simulink model "AGTF30PwrSys"  (R2021b)
settings: Solver=FixedStepDiscrete  StartTime=0.0  StopTime=MWS.In.tend  RelTol=1e-3
values from neighbouring files (symbols this model uses):
  MWS = setup_initialize(MWS,startPt,SSsolverSP)    [Setup_Simulation.m]    (also in run_AGTF30e_script.m = Setup_Simulation(inputMethod,MWS.In,filename,Mdl,SSsolverSP,)
settings Model: Creator=jlkratz  LastModifiedBy=jlkratz
settings SolverCC: ZeroCrossControl=DisableAll  AlgebraicLoopSolver=TrustRegion
settings DataIOCC: SaveOutput=off  SaveTime=off
settings DebuggingCC: SFMachineParentedDataDiag=warning
settings GRTTargetCC: CombineOutputUpdateFcns=off  MatFileLogging=off

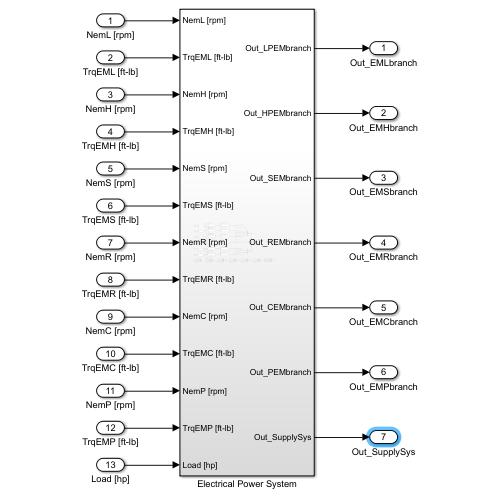
[thumbnail: Simulink's stored preview of the top-level diagram]
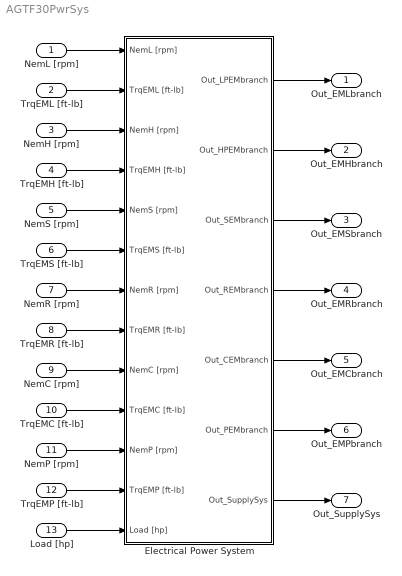
== system AGTF30PwrSys ==
  NemL [rpm] : Inport
  TrqEML [ft-lb] : Inport  Port=2
  NemH [rpm] : Inport  Port=3
  TrqEMH [ft-lb] : Inport  Port=4
  NemS [rpm] : Inport  Port=5
  TrqEMS [ft-lb] : Inport  Port=6
  NemR [rpm] : Inport  Port=7
  TrqEMR [ft-lb] : Inport  Port=8
  NemC [rpm] : Inport  Port=9
  TrqEMC [ft-lb] : Inport  Port=10
  NemP [rpm] : Inport  Port=11
  TrqEMP [ft-lb] : Inport  Port=12
  Load [hp] : Inport  Port=13
  Electrical Power System : Subsystem
  Out_EMLbranch : Outport
  Out_EMHbranch : Outport  Port=2
  Out_EMSbranch : Outport  Port=3
  Out_EMRbranch : Outport  Port=4
  Out_EMCbranch : Outport  Port=5
  Out_EMPbranch : Outport  Port=6
  Out_SupplySys : Outport  Port=7
  wires:
  NemL [rpm]/1 -> Electrical Power System/1(NemL [rpm])
  TrqEML [ft-lb]/1 -> Electrical Power System/2(TrqEML [ft-lb])
  NemH [rpm]/1 -> Electrical Power System/3(NemH [rpm])
  TrqEMH [ft-lb]/1 -> Electrical Power System/4(TrqEMH [ft-lb])
  Electrical Power System/1(Out_LPEMbranch) -> Out_EMLbranch/1
  Electrical Power System/2(Out_HPEMbranch) -> Out_EMHbranch/1
  Electrical Power System/7(Out_SupplySys) -> Out_SupplySys/1
  NemS [rpm]/1 -> Electrical Power System/5(NemS [rpm])
  TrqEMS [ft-lb]/1 -> Electrical Power System/6(TrqEMS [ft-lb])
  NemR [rpm]/1 -> Electrical Power System/7(NemR [rpm])
  TrqEMR [ft-lb]/1 -> Electrical Power System/8(TrqEMR [ft-lb])
  NemC [rpm]/1 -> Electrical Power System/9(NemC [rpm])
  TrqEMC [ft-lb]/1 -> Electrical Power System/10(TrqEMC [ft-lb])
  NemP [rpm]/1 -> Electrical Power System/11(NemP [rpm])
  TrqEMP [ft-lb]/1 -> Electrical Power System/12(TrqEMP [ft-lb])
  Load [hp]/1 -> Electrical Power System/13(Load [hp])
  Electrical Power System/3(Out_SEMbranch) -> Out_EMSbranch/1
  Electrical Power System/4(Out_REMbranch) -> Out_EMRbranch/1
  Electrical Power System/5(Out_CEMbranch) -> Out_EMCbranch/1
  Electrical Power System/6(Out_PEMbranch) -> Out_EMPbranch/1

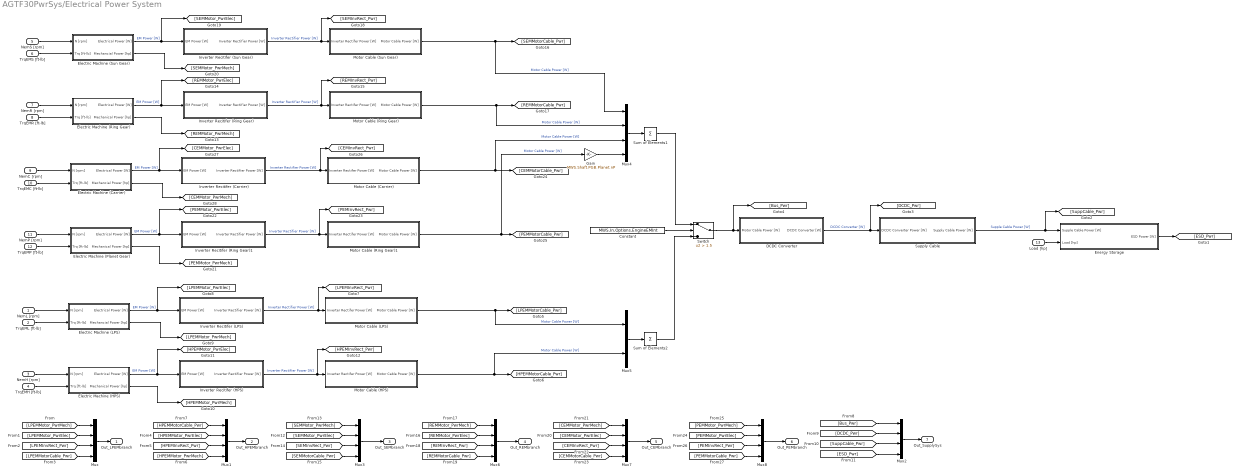
== system AGTF30PwrSys/Electrical Power System ==
  NemL [rpm] : Inport
  TrqEML [ft-lb] : Inport  Port=2
  NemH [rpm] : Inport  Port=3
  TrqEMH [ft-lb] : Inport  Port=4
  NemS [rpm] : Inport  Port=5
  TrqEMS [ft-lb] : Inport  Port=6
  NemR [rpm] : Inport  Port=7
  TrqEMR [ft-lb] : Inport  Port=8
  NemC [rpm] : Inport  Port=9
  TrqEMC [ft-lb] : Inport  Port=10
  NemP [rpm] : Inport  Port=11
  TrqEMP [ft-lb] : Inport  Port=12
  Load [hp] : Inport  Port=13
  Constant : Constant  Value=MWS.In.Options.EngineEMInt
  DCDC Converter : Subsystem
  Electric Machine (Carrier) : Subsystem
  Electric Machine (HPS) : Subsystem
  Electric Machine (LPS) : Subsystem
  Electric Machine (Planet Gear) : Subsystem
  Electric Machine (Ring Gear) : Subsystem
  Electric Machine (Sun Gear) : Subsystem
  Energy Storage : Subsystem
  Gain : Gain  Gain=MWS.Shaft.PGB.Planet.nP
  Inverter Recitifer (Carrier) : Subsystem
  Inverter Recitifer (HPS) : Subsystem
  Inverter Recitifer (LPS) : Subsystem
  Inverter Recitifer (Ring Gear) : Subsystem
  Inverter Recitifer (Ring Gear)1 : Subsystem
  Inverter Recitifer (Sun Gear) : Subsystem
  Motor Cable (Carrier) : Subsystem
  Motor Cable (HPS) : Subsystem
  Motor Cable (LPS) : Subsystem
  Motor Cable (Ring Gear) : Subsystem
  Motor Cable (Ring Gear)1 : Subsystem
  Motor Cable (Sun Gear) : Subsystem
  Mux{,1..4,6..8} (8 alike) : Mux
  Mux5 : Mux  Inputs=2
  Sum of Elements1 : Sum  Inputs=+
  Sum of Elements2 : Sum  Inputs=+
  "Supply Cable " : Subsystem
  Switch : Switch  Criteria=u2 > Threshold  Threshold=1.5
  Out_LPEMbranch : Outport
  Out_HPEMbranch : Outport  Port=2
  Out_SEMbranch : Outport  Port=3
  Out_REMbranch : Outport  Port=4
  Out_CEMbranch : Outport  Port=5
  Out_PEMbranch : Outport  Port=6
  Out_SupplySys : Outport  Port=7
  wires:
  Motor Cable (LPS)/1(Motor Cable Power [W]) -> Mux5/1, [LPEMMotorCable_Pwr]  "Motor Cable Power [W]"
  Motor Cable (HPS)/1(Motor Cable Power [W]) -> Mux5/2, [HPEMMotorCable_Pwr]  "Motor Cable Power [W]"
  Inverter Recitifer (HPS)/1(Inverter Rectifier Power [W]) -> [HPEMInvRect_Pwr], Motor Cable (HPS)/1(Inverter Rectifer Power [W])  "Inverter Rectifier Power [W]"
  [ESD_Pwr] -> Mux2/4
  "Supply Cable "/1(Supply Cable Power [W]) -> [SuppCable_Pwr], Energy Storage/1(Supple Cable Power [W])  "Supple Cable Power [W]"
  [SuppCable_Pwr] -> Mux2/3
  Electric Machine (HPS)/1(Electrical Power [W]) -> Inverter Recitifer (HPS)/1(EM Power [W]), [HPEMMotor_PwrElec]  "EM Power [W]"
  Mux2/1 -> Out_SupplySys/1
  TrqEML [ft-lb]/1 -> Electric Machine (LPS)/2(Trq [ft-lb])
  NemL [rpm]/1 -> Electric Machine (LPS)/1(N [rpm])
  Mux/1 -> Out_LPEMbranch/1
  Electric Machine (HPS)/2(Mechanical Power [hp]) -> [HPEMMotor_PwrMech]
  DCDC Converter/1(DCDC Converter [W]) -> [DCDC_Pwr], "Supply Cable "/1(DCDC Converter Power [W])  "DCDC Converter [W]"
  Inverter Recitifer (LPS)/1(Inverter Rectifier Power [W]) -> [LPEMInvRect_Pwr], Motor Cable (LPS)/1(Inverter Rectifer Power [W])  "Inverter Rectifier Power [W]"
  Switch/1 -> [Bus_Pwr], DCDC Converter/1(Motor Cable Power [W])
  NemH [rpm]/1 -> Electric Machine (HPS)/1(N [rpm])
  Electric Machine (LPS)/1(Electrical Power [W]) -> Inverter Recitifer (LPS)/1(EM Power [W]), [LPEMMotor_PwrElec]  "EM Power [W]"
  Electric Machine (LPS)/2(Mechancial Power [hp]) -> [LPEMMotor_PwrMech]
  Mux1/1 -> Out_HPEMbranch/1
  [Bus_Pwr] -> Mux2/1
  Energy Storage/1(ESD Power [W]) -> [ESD_Pwr]
  TrqEMH [ft-lb]/1 -> Electric Machine (HPS)/2(Trq [ft-lb])
  [DCDC_Pwr] -> Mux2/2
  Load [hp]/1 -> Energy Storage/2(Load [hp])
  TrqEMR [ft-lb]/1 -> Electric Machine (Ring Gear)/2(Trq [ft-lb])
  Electric Machine (Sun Gear)/2(Mechancial Power [hp]) -> [SEMMotor_PwrMech]
  Electric Machine (Sun Gear)/1(Electrical Power [W]) -> [SEMMotor_PwrElec], Inverter Recitifer (Sun Gear)/1(EM Power [W])  "EM Power [W]"
  NemR [rpm]/1 -> Electric Machine (Ring Gear)/1(N [rpm])
  Inverter Recitifer (Sun Gear)/1(Inverter Rectifier Power [W]) -> Motor Cable (Sun Gear)/1(Inverter Rectifer Power [W]), [SEMInvRect_Pwr]  "Inverter Rectifier Power [W]"
  Electric Machine (Ring Gear)/2(Mechanical Power [hp]) -> [REMMotor_PwrMech]
  NemS [rpm]/1 -> Electric Machine (Sun Gear)/1(N [rpm])
  TrqEMS [ft-lb]/1 -> Electric Machine (Sun Gear)/2(Trq [ft-lb])
  Electric Machine (Ring Gear)/1(Electrical Power [W]) -> [REMMotor_PwrElec], Inverter Recitifer (Ring Gear)/1(EM Power [W])  "EM Power [W]"
  Inverter Recitifer (Ring Gear)/1(Inverter Rectifier Power [W]) -> Motor Cable (Ring Gear)/1(Inverter Rectifer Power [W]), [REMInvRect_Pwr]  "Inverter Rectifier Power [W]"
  Motor Cable (Ring Gear)/1(Motor Cable Power [W]) -> Mux4/2, [REMMotorCable_Pwr]  "Motor Cable Power [W]"
  Motor Cable (Sun Gear)/1(Motor Cable Power [W]) -> [SEMMotorCable_Pwr], Mux4/1  "Motor Cable Power [W]"
  Motor Cable (Carrier)/1(Motor Cable Power [W]) -> Mux4/3, [CEMMotorCable_Pwr]  "Motor Cable Power [W]"
  Motor Cable (Ring Gear)1/1(Motor Cable Power [W]) -> [PEMMotorCable_Pwr], Gain/1  "Motor Cable Power [W]"
  Inverter Recitifer (Ring Gear)1/1(Inverter Rectifier Power [W]) -> [PEMInvRect_Pwr], Motor Cable (Ring Gear)1/1(Inverter Rectifer Power [W])  "Inverter Rectifier Power [W]"
  Electric Machine (Planet Gear)/1(Electrical Power [W]) -> Inverter Recitifer (Ring Gear)1/1(EM Power [W]), [PEMMotor_PwrElec]  "EM Power [W]"
  TrqEMC [ft-lb]/1 -> Electric Machine (Carrier)/2(Trq [ft-lb])
  NemC [rpm]/1 -> Electric Machine (Carrier)/1(N [rpm])
  Electric Machine (Planet Gear)/2(Mechanical Power [hp]) -> [PEMMotor_PwrMech]
  Inverter Recitifer (Carrier)/1(Inverter Rectifier Power [W]) -> [CEMInvRect_Pwr], Motor Cable (Carrier)/1(Inverter Rectifer Power [W])  "Inverter Rectifier Power [W]"
  NemP [rpm]/1 -> Electric Machine (Planet Gear)/1(N [rpm])
  Electric Machine (Carrier)/1(Electrical Power [W]) -> Inverter Recitifer (Carrier)/1(EM Power [W]), [CEMMotor_PwrElec]  "EM Power [W]"
  Electric Machine (Carrier)/2(Mechancial Power [hp]) -> [CEMMotor_PwrMech]
  TrqEMP [ft-lb]/1 -> Electric Machine (Planet Gear)/2(Trq [ft-lb])
  Mux4/1 -> Sum of Elements1/1
  Mux5/1 -> Sum of Elements2/1
  Sum of Elements1/1 -> Switch/1
  Sum of Elements2/1 -> Switch/3
  Constant/1 -> Switch/2
  [SEMMotor_PwrMech] -> Mux3/1
  [SEMMotor_PwrElec] -> Mux3/2
  [SEMInvRect_Pwr] -> Mux3/3
  [SEMMotorCable_Pwr] -> Mux3/4
  [LPEMMotor_PwrMech] -> Mux/1
  [LPEMMotor_PwrElec] -> Mux/2
  [LPEMInvRect_Pwr] -> Mux/3
  [LPEMMotorCable_Pwr] -> Mux/4
  [HPEMMotor_PwrElec] -> Mux1/2
  [HPEMInvRect_Pwr] -> Mux1/3
  [HPEMMotor_PwrMech] -> Mux1/4
  [HPEMMotorCable_Pwr] -> Mux1/1
  Mux3/1 -> Out_SEMbranch/1
  Mux6/1 -> Out_REMbranch/1
  [REMMotorCable_Pwr] -> Mux6/4
  [REMInvRect_Pwr] -> Mux6/3
  [REMMotor_PwrElec] -> Mux6/2
  [REMMotor_PwrMech] -> Mux6/1
  [PEMMotor_PwrMech] -> Mux8/1
  [PEMMotor_PwrElec] -> Mux8/2
  [PEMInvRect_Pwr] -> Mux8/3
  [PEMMotorCable_Pwr] -> Mux8/4
  Mux8/1 -> Out_PEMbranch/1
  Mux7/1 -> Out_CEMbranch/1
  [CEMMotorCable_Pwr] -> Mux7/4
  [CEMInvRect_Pwr] -> Mux7/3
  [CEMMotor_PwrElec] -> Mux7/2
  [CEMMotor_PwrMech] -> Mux7/1
  Gain/1 -> Mux4/4

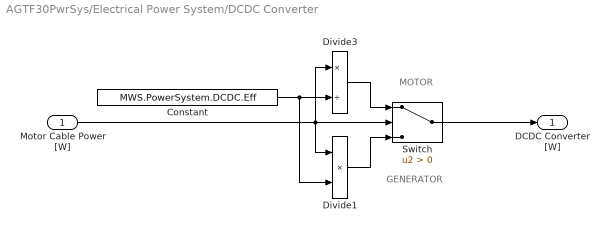
== system AGTF30PwrSys/Electrical Power System/DCDC Converter ==
  note: GENERATOR
  note: MOTOR
  Motor Cable Power [W] : Inport
  Constant : Constant  Value=MWS.PowerSystem.DCDC.Eff
  Divide1 : Product  Inputs=**
  Divide3 : Product  Inputs=*/
  Switch : Switch  Criteria=u2 > Threshold
  DCDC Converter [W] : Outport
  wires:
  Constant/1 -> Divide1/2, Divide3/2
  Switch/1 -> DCDC Converter [W]/1
  Divide3/1 -> Switch/1
  Divide1/1 -> Switch/3
  Motor Cable Power [W]/1 -> Divide3/1, Divide1/1, Switch/2

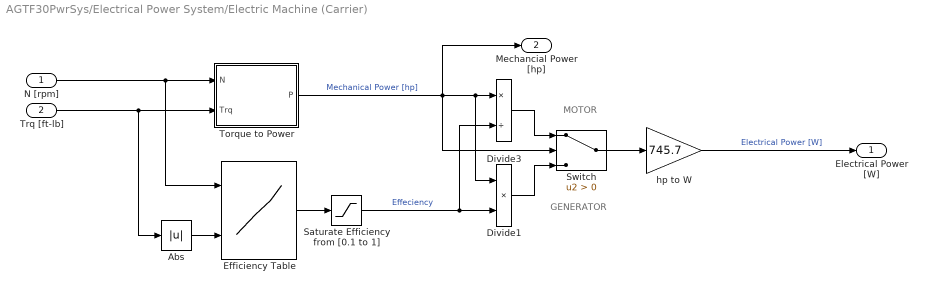
== system AGTF30PwrSys/Electrical Power System/Electric Machine (Carrier) ==
  note: MOTOR
  note: GENERATOR
  N [rpm] : Inport
  Trq [ft-lb] : Inport  Port=2
  Abs : Abs
  Divide1 : Product  Inputs=**
  Divide3 : Product  Inputs=*/
  Efficiency Table : Lookup_n-D  BreakpointsForDimension1=MWS.PowerSystem.EMS.Speed  BreakpointsForDimension2=MWS.PowerSystem.EMS.Torque  Table=MWS.PowerSystem.EMS.Eff  ExtrapMethod=Clip  InternalRulePriority=Speed  RndMeth=Simplest  InputSameDT=on
      settings: InputPortMap=u0,u1
  Saturate Efficiency from [0.1 to 1] : Saturate  UpperLimit=1  LowerLimit=0.1
  Switch : Switch  Criteria=u2 > Threshold
  Torque to Power : Subsystem
  hp to W : Gain  Gain=745.7
  Electrical Power [W] : Outport
  Mechancial Power [hp] : Outport  Port=2
  wires:
  Switch/1 -> hp to W/1
  Saturate Efficiency from [0.1 to 1]/1 -> Divide3/2, Divide1/2  "Effeciency"
  Torque to Power/1(P) -> Mechancial Power [hp]/1, Switch/2, Divide1/1, Divide3/1  "Mechanical Power [hp]"
  Divide1/1 -> Switch/3
  N [rpm]/1 -> Efficiency Table/1, Torque to Power/1(N)
  Efficiency Table/1 -> Saturate Efficiency from [0.1 to 1]/1
  Trq [ft-lb]/1 -> Abs/1, Torque to Power/2(Trq)
  Abs/1 -> Efficiency Table/2
  Divide3/1 -> Switch/1
  hp to W/1 -> Electrical Power [W]/1  "Electrical Power [W]"

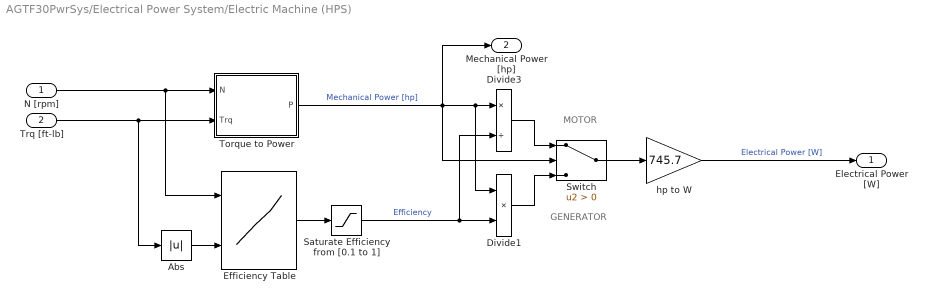
== system AGTF30PwrSys/Electrical Power System/Electric Machine (HPS) ==
  note: GENERATOR
  note: MOTOR
  N [rpm] : Inport
  Trq [ft-lb] : Inport  Port=2
  Abs : Abs
  Divide1 : Product  Inputs=**
  Divide3 : Product  Inputs=*/
  Efficiency Table : Lookup_n-D  BreakpointsForDimension1=MWS.PowerSystem.EMH.Speed  BreakpointsForDimension2=MWS.PowerSystem.EMH.Torque  Table=MWS.PowerSystem.EMH.Eff  ExtrapMethod=Clip  InternalRulePriority=Speed  RndMeth=Simplest  InputSameDT=on
      settings: InputPortMap=u0,u1
  Saturate Efficiency from [0.1 to 1] : Saturate  UpperLimit=1  LowerLimit=0.1
  Switch : Switch  Criteria=u2 > Threshold
  Torque to Power : Subsystem
  hp to W : Gain  Gain=745.7
  Electrical Power [W] : Outport
  Mechanical Power [hp] : Outport  Port=2
  wires:
  hp to W/1 -> Electrical Power [W]/1  "Electrical Power [W]"
  Divide3/1 -> Switch/1
  Abs/1 -> Efficiency Table/2
  Trq [ft-lb]/1 -> Torque to Power/2(Trq), Abs/1
  Efficiency Table/1 -> Saturate Efficiency from [0.1 to 1]/1
  N [rpm]/1 -> Torque to Power/1(N), Efficiency Table/1
  Divide1/1 -> Switch/3
  Torque to Power/1(P) -> Mechanical Power [hp]/1, Divide3/1, Divide1/1, Switch/2  "Mechanical Power [hp]"
  Saturate Efficiency from [0.1 to 1]/1 -> Divide1/2, Divide3/2  "Efficiency"
  Switch/1 -> hp to W/1

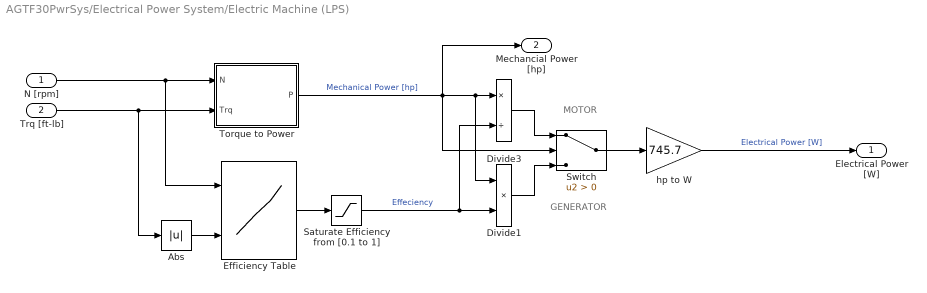
== system AGTF30PwrSys/Electrical Power System/Electric Machine (LPS) ==
  note: MOTOR
  note: GENERATOR
  N [rpm] : Inport
  Trq [ft-lb] : Inport  Port=2
  Abs : Abs
  Divide1 : Product  Inputs=**
  Divide3 : Product  Inputs=*/
  Efficiency Table : Lookup_n-D  BreakpointsForDimension1=MWS.PowerSystem.EML.Speed  BreakpointsForDimension2=MWS.PowerSystem.EML.Torque  Table=MWS.PowerSystem.EML.Eff  ExtrapMethod=Clip  InternalRulePriority=Speed  RndMeth=Simplest  InputSameDT=on
      settings: InputPortMap=u0,u1
  Saturate Efficiency from [0.1 to 1] : Saturate  UpperLimit=1  LowerLimit=0.1
  Switch : Switch  Criteria=u2 > Threshold
  Torque to Power : Subsystem
  hp to W : Gain  Gain=745.7
  Electrical Power [W] : Outport
  Mechancial Power [hp] : Outport  Port=2
  wires:
  Switch/1 -> hp to W/1
  Saturate Efficiency from [0.1 to 1]/1 -> Divide3/2, Divide1/2  "Effeciency"
  Torque to Power/1(P) -> Mechancial Power [hp]/1, Switch/2, Divide1/1, Divide3/1  "Mechanical Power [hp]"
  Divide1/1 -> Switch/3
  N [rpm]/1 -> Efficiency Table/1, Torque to Power/1(N)
  Efficiency Table/1 -> Saturate Efficiency from [0.1 to 1]/1
  Trq [ft-lb]/1 -> Abs/1, Torque to Power/2(Trq)
  Abs/1 -> Efficiency Table/2
  Divide3/1 -> Switch/1
  hp to W/1 -> Electrical Power [W]/1  "Electrical Power [W]"

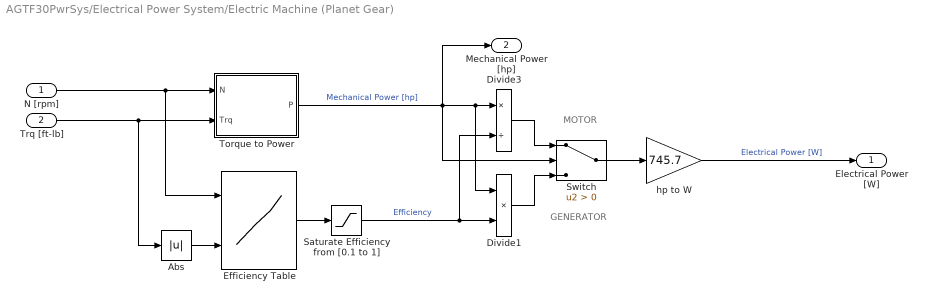
== system AGTF30PwrSys/Electrical Power System/Electric Machine (Planet Gear) ==
  note: GENERATOR
  note: MOTOR
  N [rpm] : Inport
  Trq [ft-lb] : Inport  Port=2
  Abs : Abs
  Divide1 : Product  Inputs=**
  Divide3 : Product  Inputs=*/
  Efficiency Table : Lookup_n-D  BreakpointsForDimension1=MWS.PowerSystem.EMR.Speed  BreakpointsForDimension2=MWS.PowerSystem.EMR.Torque  Table=MWS.PowerSystem.EMR.Eff  ExtrapMethod=Clip  InternalRulePriority=Speed  RndMeth=Simplest  InputSameDT=on
      settings: InputPortMap=u0,u1
  Saturate Efficiency from [0.1 to 1] : Saturate  UpperLimit=1  LowerLimit=0.1
  Switch : Switch  Criteria=u2 > Threshold
  Torque to Power : Subsystem
  hp to W : Gain  Gain=745.7
  Electrical Power [W] : Outport
  Mechanical Power [hp] : Outport  Port=2
  wires:
  hp to W/1 -> Electrical Power [W]/1  "Electrical Power [W]"
  Divide3/1 -> Switch/1
  Abs/1 -> Efficiency Table/2
  Trq [ft-lb]/1 -> Torque to Power/2(Trq), Abs/1
  Efficiency Table/1 -> Saturate Efficiency from [0.1 to 1]/1
  N [rpm]/1 -> Torque to Power/1(N), Efficiency Table/1
  Divide1/1 -> Switch/3
  Torque to Power/1(P) -> Mechanical Power [hp]/1, Divide3/1, Divide1/1, Switch/2  "Mechanical Power [hp]"
  Saturate Efficiency from [0.1 to 1]/1 -> Divide1/2, Divide3/2  "Efficiency"
  Switch/1 -> hp to W/1

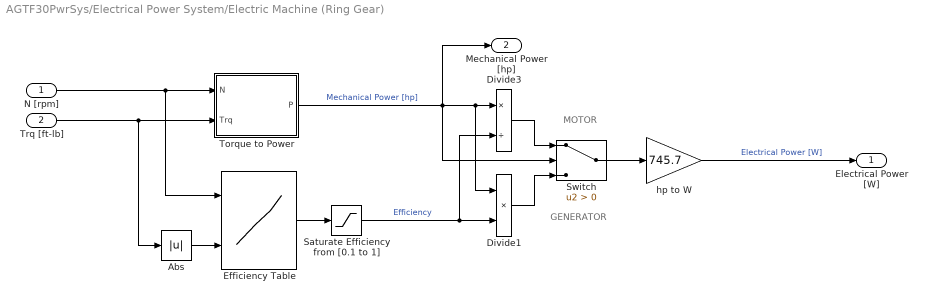
== system AGTF30PwrSys/Electrical Power System/Electric Machine (Ring Gear) ==
  note: MOTOR
  note: GENERATOR
  N [rpm] : Inport
  Trq [ft-lb] : Inport  Port=2
  Abs : Abs
  Divide1 : Product  Inputs=**
  Divide3 : Product  Inputs=*/
  Efficiency Table : Lookup_n-D  BreakpointsForDimension1=MWS.PowerSystem.EMR.Speed  BreakpointsForDimension2=MWS.PowerSystem.EMR.Torque  Table=MWS.PowerSystem.EMR.Eff  ExtrapMethod=Clip  InternalRulePriority=Speed  RndMeth=Simplest  InputSameDT=on
      settings: InputPortMap=u0,u1
  Saturate Efficiency from [0.1 to 1] : Saturate  UpperLimit=1  LowerLimit=0.1
  Switch : Switch  Criteria=u2 > Threshold
  Torque to Power : Subsystem
  hp to W : Gain  Gain=745.7
  Electrical Power [W] : Outport
  Mechanical Power [hp] : Outport  Port=2
  wires:
  Switch/1 -> hp to W/1
  Saturate Efficiency from [0.1 to 1]/1 -> Divide3/2, Divide1/2  "Efficiency"
  Torque to Power/1(P) -> Switch/2, Divide1/1, Divide3/1, Mechanical Power [hp]/1  "Mechanical Power [hp]"
  Divide1/1 -> Switch/3
  N [rpm]/1 -> Efficiency Table/1, Torque to Power/1(N)
  Efficiency Table/1 -> Saturate Efficiency from [0.1 to 1]/1
  Trq [ft-lb]/1 -> Abs/1, Torque to Power/2(Trq)
  Abs/1 -> Efficiency Table/2
  Divide3/1 -> Switch/1
  hp to W/1 -> Electrical Power [W]/1  "Electrical Power [W]"

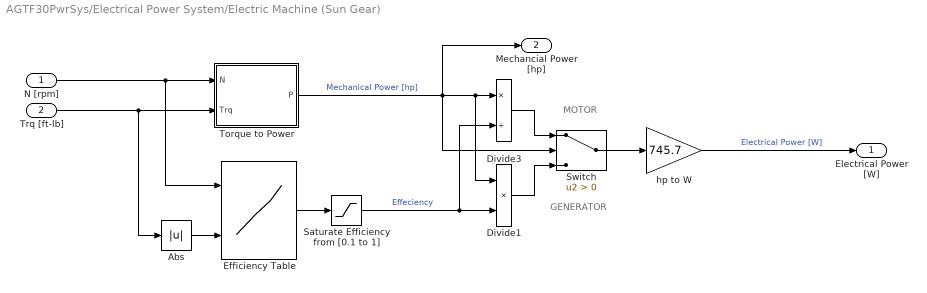
== system AGTF30PwrSys/Electrical Power System/Electric Machine (Sun Gear) ==
  note: GENERATOR
  note: MOTOR
  N [rpm] : Inport
  Trq [ft-lb] : Inport  Port=2
  Abs : Abs
  Divide1 : Product  Inputs=**
  Divide3 : Product  Inputs=*/
  Efficiency Table : Lookup_n-D  BreakpointsForDimension1=MWS.PowerSystem.EMS.Speed  BreakpointsForDimension2=MWS.PowerSystem.EMS.Torque  Table=MWS.PowerSystem.EMS.Eff  ExtrapMethod=Clip  InternalRulePriority=Speed  RndMeth=Simplest  InputSameDT=on
      settings: InputPortMap=u0,u1
  Saturate Efficiency from [0.1 to 1] : Saturate  UpperLimit=1  LowerLimit=0.1
  Switch : Switch  Criteria=u2 > Threshold
  Torque to Power : Subsystem
  hp to W : Gain  Gain=745.7
  Electrical Power [W] : Outport
  Mechancial Power [hp] : Outport  Port=2
  wires:
  hp to W/1 -> Electrical Power [W]/1  "Electrical Power [W]"
  Divide3/1 -> Switch/1
  Abs/1 -> Efficiency Table/2
  Trq [ft-lb]/1 -> Torque to Power/2(Trq), Abs/1
  Efficiency Table/1 -> Saturate Efficiency from [0.1 to 1]/1
  N [rpm]/1 -> Torque to Power/1(N), Efficiency Table/1
  Divide1/1 -> Switch/3
  Torque to Power/1(P) -> Divide3/1, Divide1/1, Switch/2, Mechancial Power [hp]/1  "Mechanical Power [hp]"
  Saturate Efficiency from [0.1 to 1]/1 -> Divide1/2, Divide3/2  "Effeciency"
  Switch/1 -> hp to W/1

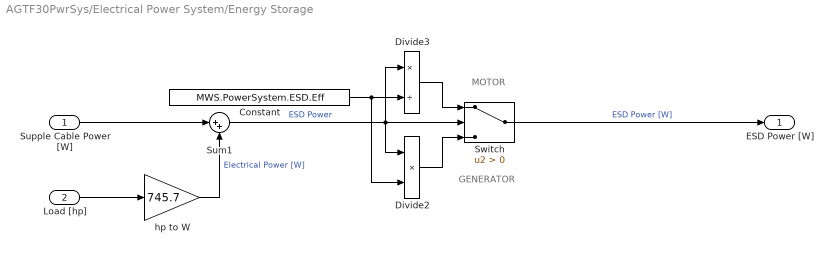
== system AGTF30PwrSys/Electrical Power System/Energy Storage ==
  note: MOTOR
  note: GENERATOR
  Supple Cable Power [W] : Inport
  Load [hp] : Inport  Port=2
  Constant : Constant  Value=MWS.PowerSystem.ESD.Eff
  Divide2 : Product  Inputs=**
  Divide3 : Product  Inputs=*/
  Sum1 : Sum  Inputs=|++
  Switch : Switch  Criteria=u2 > Threshold
  hp to W : Gain  Gain=745.7
  ESD Power [W] : Outport
  wires:
  Switch/1 -> ESD Power [W]/1  "ESD Power [W]"
  Supple Cable Power [W]/1 -> Sum1/1
  Constant/1 -> Divide3/2, Divide2/2
  Divide3/1 -> Switch/1
  Divide2/1 -> Switch/3
  hp to W/1 -> Sum1/2  "Electrical Power [W]"
  Sum1/1 -> Divide3/1, Divide2/1, Switch/2  "ESD Power"
  Load [hp]/1 -> hp to W/1

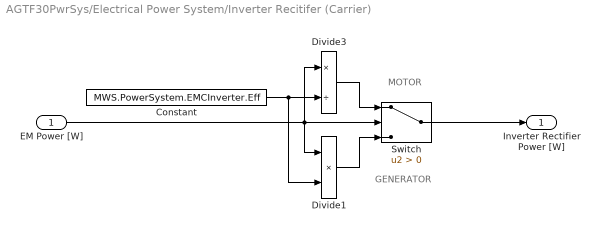
== system AGTF30PwrSys/Electrical Power System/Inverter Recitifer (Carrier) ==
  note: GENERATOR
  note: MOTOR
  EM Power [W] : Inport
  Constant : Constant  Value=MWS.PowerSystem.EMCInverter.Eff
  Divide1 : Product  Inputs=**
  Divide3 : Product  Inputs=*/
  Switch : Switch  Criteria=u2 > Threshold
  Inverter Rectifier Power [W] : Outport
  wires:
  Constant/1 -> Divide1/2, Divide3/2
  Switch/1 -> Inverter Rectifier Power [W]/1
  Divide3/1 -> Switch/1
  Divide1/1 -> Switch/3
  EM Power [W]/1 -> Divide3/1, Divide1/1, Switch/2

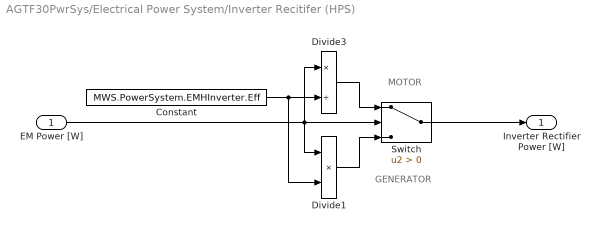
== system AGTF30PwrSys/Electrical Power System/Inverter Recitifer (HPS) ==
  note: MOTOR
  note: GENERATOR
  EM Power [W] : Inport
  Constant : Constant  Value=MWS.PowerSystem.EMHInverter.Eff
  Divide1 : Product  Inputs=**
  Divide3 : Product  Inputs=*/
  Switch : Switch  Criteria=u2 > Threshold
  Inverter Rectifier Power [W] : Outport
  wires:
  EM Power [W]/1 -> Divide3/1, Switch/2, Divide1/1
  Divide1/1 -> Switch/3
  Divide3/1 -> Switch/1
  Switch/1 -> Inverter Rectifier Power [W]/1
  Constant/1 -> Divide3/2, Divide1/2

== system AGTF30PwrSys/Electrical Power System/Inverter Recitifer (LPS) ==
  note: GENERATOR
  note: MOTOR
  EM Power [W] : Inport
  Constant : Constant  Value=MWS.PowerSystem.EMLInverter.Eff
  Divide1 : Product  Inputs=**
  Divide3 : Product  Inputs=*/
  Switch : Switch  Criteria=u2 > Threshold
  Inverter Rectifier Power [W] : Outport
  wires:
  Constant/1 -> Divide1/2, Divide3/2
  Switch/1 -> Inverter Rectifier Power [W]/1
  Divide3/1 -> Switch/1
  Divide1/1 -> Switch/3
  EM Power [W]/1 -> Divide3/1, Divide1/1, Switch/2

== system AGTF30PwrSys/Electrical Power System/Inverter Recitifer (Ring Gear) ==
  note: GENERATOR
  note: MOTOR
  EM Power [W] : Inport
  Constant : Constant  Value=MWS.PowerSystem.EMRInverter.Eff
  Divide1 : Product  Inputs=**
  Divide3 : Product  Inputs=*/
  Switch : Switch  Criteria=u2 > Threshold
  Inverter Rectifier Power [W] : Outport
  wires:
  Constant/1 -> Divide1/2, Divide3/2
  Switch/1 -> Inverter Rectifier Power [W]/1
  Divide3/1 -> Switch/1
  Divide1/1 -> Switch/3
  EM Power [W]/1 -> Divide1/1, Switch/2, Divide3/1

== system AGTF30PwrSys/Electrical Power System/Inverter Recitifer (Ring Gear)1 ==
  note: MOTOR
  note: GENERATOR
  EM Power [W] : Inport
  Constant : Constant  Value=MWS.PowerSystem.EMPInverter.Eff
  Divide1 : Product  Inputs=**
  Divide3 : Product  Inputs=*/
  Switch : Switch  Criteria=u2 > Threshold
  Inverter Rectifier Power [W] : Outport
  wires:
  EM Power [W]/1 -> Divide3/1, Switch/2, Divide1/1
  Divide1/1 -> Switch/3
  Divide3/1 -> Switch/1
  Switch/1 -> Inverter Rectifier Power [W]/1
  Constant/1 -> Divide3/2, Divide1/2

== system AGTF30PwrSys/Electrical Power System/Inverter Recitifer (Sun Gear) ==
  note: MOTOR
  note: GENERATOR
  EM Power [W] : Inport
  Constant : Constant  Value=MWS.PowerSystem.EMSInverter.Eff
  Divide1 : Product  Inputs=**
  Divide3 : Product  Inputs=*/
  Switch : Switch  Criteria=u2 > Threshold
  Inverter Rectifier Power [W] : Outport
  wires:
  EM Power [W]/1 -> Switch/2, Divide1/1, Divide3/1
  Divide1/1 -> Switch/3
  Divide3/1 -> Switch/1
  Switch/1 -> Inverter Rectifier Power [W]/1
  Constant/1 -> Divide3/2, Divide1/2

== system AGTF30PwrSys/Electrical Power System/Motor Cable (Carrier) ==
  note: MOTOR
  note: GENERATOR
  Inverter Rectifer Power [W] : Inport
  Constant : Constant  Value=MWS.PowerSystem.MotorCable.Eff
  Divide1 : Product  Inputs=**
  Divide3 : Product  Inputs=*/
  Switch : Switch  Criteria=u2 > Threshold
  Motor Cable Power [W] : Outport
  wires:
  Inverter Rectifer Power [W]/1 -> Divide3/1, Switch/2, Divide1/1
  Divide1/1 -> Switch/3
  Divide3/1 -> Switch/1
  Switch/1 -> Motor Cable Power [W]/1
  Constant/1 -> Divide3/2, Divide1/2

== system AGTF30PwrSys/Electrical Power System/Motor Cable (HPS) ==
  note: GENERATOR
  note: MOTOR
  Inverter Rectifer Power [W] : Inport
  Constant : Constant  Value=MWS.PowerSystem.MotorCable.Eff
  Divide1 : Product  Inputs=**
  Divide3 : Product  Inputs=*/
  Switch : Switch  Criteria=u2 > Threshold
  Motor Cable Power [W] : Outport
  wires:
  Constant/1 -> Divide1/2, Divide3/2
  Switch/1 -> Motor Cable Power [W]/1
  Divide3/1 -> Switch/1
  Divide1/1 -> Switch/3
  Inverter Rectifer Power [W]/1 -> Divide1/1, Divide3/1, Switch/2

== system AGTF30PwrSys/Electrical Power System/Motor Cable (LPS) ==
  note: MOTOR
  note: GENERATOR
  Inverter Rectifer Power [W] : Inport
  Constant : Constant  Value=MWS.PowerSystem.MotorCable.Eff
  Divide1 : Product  Inputs=**
  Divide3 : Product  Inputs=*/
  Switch : Switch  Criteria=u2 > Threshold
  Motor Cable Power [W] : Outport
  wires:
  Inverter Rectifer Power [W]/1 -> Divide3/1, Switch/2, Divide1/1
  Divide1/1 -> Switch/3
  Divide3/1 -> Switch/1
  Switch/1 -> Motor Cable Power [W]/1
  Constant/1 -> Divide3/2, Divide1/2

== system AGTF30PwrSys/Electrical Power System/Motor Cable (Ring Gear) ==
  note: MOTOR
  note: GENERATOR
  Inverter Rectifer Power [W] : Inport
  Constant : Constant  Value=MWS.PowerSystem.MotorCable.Eff
  Divide1 : Product  Inputs=**
  Divide3 : Product  Inputs=*/
  Switch : Switch  Criteria=u2 > Threshold
  Motor Cable Power [W] : Outport
  wires:
  Inverter Rectifer Power [W]/1 -> Switch/2, Divide3/1, Divide1/1
  Divide1/1 -> Switch/3
  Divide3/1 -> Switch/1
  Switch/1 -> Motor Cable Power [W]/1
  Constant/1 -> Divide3/2, Divide1/2

== system AGTF30PwrSys/Electrical Power System/Motor Cable (Ring Gear)1 ==
  note: GENERATOR
  note: MOTOR
  Inverter Rectifer Power [W] : Inport
  Constant : Constant  Value=MWS.PowerSystem.MotorCable.Eff
  Divide1 : Product  Inputs=**
  Divide3 : Product  Inputs=*/
  Switch : Switch  Criteria=u2 > Threshold
  Motor Cable Power [W] : Outport
  wires:
  Constant/1 -> Divide1/2, Divide3/2
  Switch/1 -> Motor Cable Power [W]/1
  Divide3/1 -> Switch/1
  Divide1/1 -> Switch/3
  Inverter Rectifer Power [W]/1 -> Divide1/1, Divide3/1, Switch/2

== system AGTF30PwrSys/Electrical Power System/Motor Cable (Sun Gear) ==
  note: GENERATOR
  note: MOTOR
  Inverter Rectifer Power [W] : Inport
  Constant : Constant  Value=MWS.PowerSystem.MotorCable.Eff
  Divide1 : Product  Inputs=**
  Divide3 : Product  Inputs=*/
  Switch : Switch  Criteria=u2 > Threshold
  Motor Cable Power [W] : Outport
  wires:
  Constant/1 -> Divide1/2, Divide3/2
  Switch/1 -> Motor Cable Power [W]/1
  Divide3/1 -> Switch/1
  Divide1/1 -> Switch/3
  Inverter Rectifer Power [W]/1 -> Divide1/1, Switch/2, Divide3/1

== system AGTF30PwrSys/Electrical Power System/Supply Cable  ==
  note: MOTOR
  note: GENERATOR
  DCDC Converter Power [W] : Inport
  Constant : Constant  Value=MWS.PowerSystem.SupplyCable.Eff
  Divide1 : Product  Inputs=**
  Divide3 : Product  Inputs=*/
  Switch : Switch  Criteria=u2 > Threshold
  Supply Cable Power [W] : Outport
  wires:
  DCDC Converter Power [W]/1 -> Divide3/1, Switch/2, Divide1/1
  Divide1/1 -> Switch/3
  Divide3/1 -> Switch/1
  Switch/1 -> Supply Cable Power [W]/1
  Constant/1 -> Divide3/2, Divide1/2

== system AGTF30PwrSys/Electrical Power System/Electric Machine (Carrier)/Torque to Power ==
  N : Inport
  Trq : Inport  Port=2
  Divide : Product  Inputs=**
  Gain : Gain  Gain=1/5252.113
  P : Outport
  wires:
  Divide/1 -> Gain/1
  Gain/1 -> P/1  "Mechanical Power"
  Trq/1 -> Divide/2
  N/1 -> Divide/1

== system AGTF30PwrSys/Electrical Power System/Electric Machine (HPS)/Torque to Power ==
  N : Inport
  Trq : Inport  Port=2
  Divide : Product  Inputs=**
  Gain : Gain  Gain=1/5252.113
  P : Outport
  wires:
  N/1 -> Divide/1
  Trq/1 -> Divide/2
  Gain/1 -> P/1  "Mechanical Power"
  Divide/1 -> Gain/1

== system AGTF30PwrSys/Electrical Power System/Electric Machine (LPS)/Torque to Power ==
  N : Inport
  Trq : Inport  Port=2
  Divide : Product  Inputs=**
  Gain : Gain  Gain=1/5252.113
  P : Outport
  wires:
  Divide/1 -> Gain/1
  Gain/1 -> P/1  "Mechanical Power"
  Trq/1 -> Divide/2
  N/1 -> Divide/1

== system AGTF30PwrSys/Electrical Power System/Electric Machine (Planet Gear)/Torque to Power ==
  N : Inport
  Trq : Inport  Port=2
  Divide : Product  Inputs=**
  Gain : Gain  Gain=1/5252.113
  P : Outport
  wires:
  N/1 -> Divide/1
  Trq/1 -> Divide/2
  Gain/1 -> P/1  "Mechanical Power"
  Divide/1 -> Gain/1

== system AGTF30PwrSys/Electrical Power System/Electric Machine (Ring Gear)/Torque to Power ==
  N : Inport
  Trq : Inport  Port=2
  Divide : Product  Inputs=**
  Gain : Gain  Gain=1/5252.113
  P : Outport
  wires:
  Divide/1 -> Gain/1
  Gain/1 -> P/1  "Mechanical Power"
  Trq/1 -> Divide/2
  N/1 -> Divide/1

== system AGTF30PwrSys/Electrical Power System/Electric Machine (Sun Gear)/Torque to Power ==
  N : Inport
  Trq : Inport  Port=2
  Divide : Product  Inputs=**
  Gain : Gain  Gain=1/5252.113
  P : Outport
  wires:
  N/1 -> Divide/1
  Trq/1 -> Divide/2
  Gain/1 -> P/1  "Mechanical Power"
  Divide/1 -> Gain/1
